simulink model "cocheaArriba"  (R2024a)
settings: Solver=VariableStepAuto  StartTime=0.0  StopTime=365*4  RelTol=1e-3
settings Model: Creator=gerar  LastModifiedBy=gerar

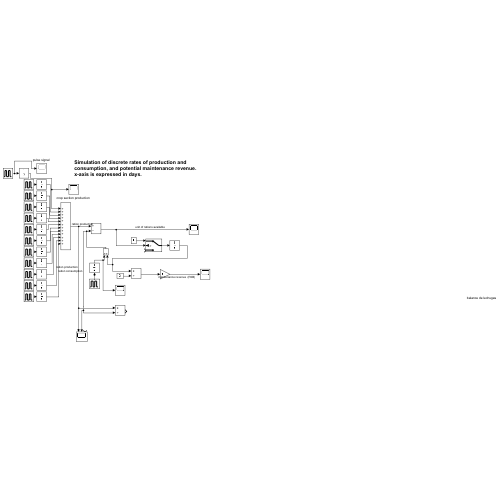
[thumbnail: Simulink's stored preview of the top-level diagram]
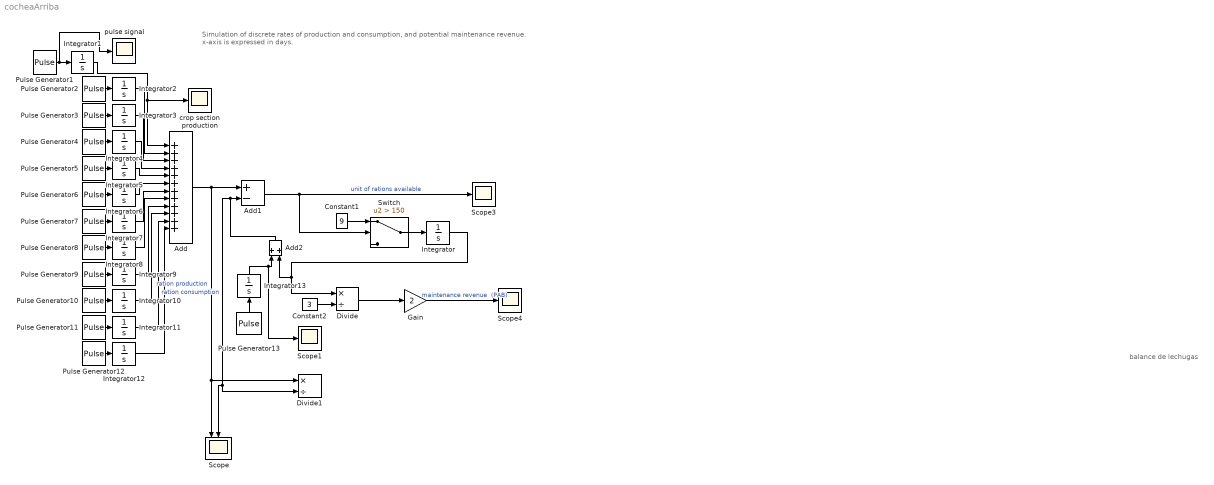
== system cocheaArriba ==
  note: Simulation of discrete rates of production and consumption, and potential maintenance revenue. x-axis is expressed in days.
  note: balance de lechugas
  Add : Sum  Inputs=++++++++++++
  Add1 : Sum  Inputs=+-
  Add2 : Sum
  Constant1 : Constant  Value=9
  Constant2 : Constant  Value=3
  Divide : Product  Inputs=*/
  Divide1 : Product  Inputs=*/
  Gain : Gain  Gain=2
  Integrator{,1..13} (14 alike) : Integrator
  Pulse Generator1 : DiscretePulseGenerator  PulseType=Time based  Amplitude=31  Period=37  PulseWidth=2.703  PhaseDelay=37
  Pulse Generator10 : DiscretePulseGenerator  PulseType=Time based  Amplitude=31  Period=37  PulseWidth=2.703  PhaseDelay=21+37
  Pulse Generator11 : DiscretePulseGenerator  PulseType=Time based  Amplitude=31  Period=37  PulseWidth=2.703  PhaseDelay=23+37
  Pulse Generator12 : DiscretePulseGenerator  PulseType=Time based  Amplitude=31  Period=37  PulseWidth=2.703  PhaseDelay=25+37
  Pulse Generator13 : DiscretePulseGenerator  PulseType=Time based  Amplitude=65  Period=7  PulseWidth=14.3  PhaseDelay=74
  Pulse Generator2 : DiscretePulseGenerator  PulseType=Time based  Amplitude=31  Period=37  PulseWidth=2.703  PhaseDelay=2+37
  Pulse Generator3 : DiscretePulseGenerator  PulseType=Time based  Amplitude=31  Period=37  PulseWidth=2.703  PhaseDelay=4+37
  Pulse Generator4 : DiscretePulseGenerator  PulseType=Time based  Amplitude=31  Period=37  PulseWidth=2.703  PhaseDelay=7+37
  Pulse Generator5 : DiscretePulseGenerator  PulseType=Time based  Amplitude=31  Period=37  PulseWidth=2.703  PhaseDelay=9+37
  Pulse Generator6 : DiscretePulseGenerator  PulseType=Time based  Amplitude=31  Period=37  PulseWidth=2.703  PhaseDelay=11+37
  Pulse Generator7 : DiscretePulseGenerator  PulseType=Time based  Amplitude=31  Period=37  PulseWidth=2.703  PhaseDelay=14+37
  Pulse Generator8 : DiscretePulseGenerator  PulseType=Time based  Amplitude=31  Period=37  PulseWidth=2.703  PhaseDelay=16+37
  Pulse Generator9 : DiscretePulseGenerator  PulseType=Time based  Amplitude=31  Period=37  PulseWidth=2.703  PhaseDelay=18+37
  Scope : Scope  NumInputPorts=3
  Scope1 : Scope
  Scope3 : Scope
  Scope4 : Scope
  Switch : Switch  Criteria=u2 > Threshold  Threshold=150  SaturateOnIntegerOverflow=off  InputSameDT=off
  "crop section production " : Scope
  "pulse signal " : Scope
  wires:
  Pulse Generator13/1 -> Integrator13/1
  Switch/1 -> Integrator/1
  Integrator/1 -> Add2/2, Divide/1
  Constant2/1 -> Divide/2
  Divide/1 -> Gain/1
  Gain/1 -> Scope4/1  "maintenance revenue  (PAB)"
  Pulse Generator1/1 -> "pulse signal "/1, Integrator1/1
  Pulse Generator2/1 -> Integrator2/1
  Pulse Generator3/1 -> Integrator3/1
  Pulse Generator4/1 -> Integrator4/1
  Pulse Generator5/1 -> Integrator5/1
  Pulse Generator6/1 -> Integrator6/1
  Pulse Generator7/1 -> Integrator7/1
  Pulse Generator8/1 -> Integrator8/1
  Pulse Generator9/1 -> Integrator9/1
  Pulse Generator10/1 -> Integrator10/1
  Pulse Generator11/1 -> Integrator11/1
  Pulse Generator12/1 -> Integrator12/1
  Integrator12/1 -> Add/12
  Integrator11/1 -> Add/11
  Integrator10/1 -> Add/10
  Integrator9/1 -> Add/9
  Integrator8/1 -> Add/8
  Integrator7/1 -> Add/7
  Integrator6/1 -> Add/6
  Integrator5/1 -> Add/5
  Integrator4/1 -> Add/4
  Integrator3/1 -> Add/3
  Integrator2/1 -> Add/2
  Integrator1/1 -> Add/1, "crop section production "/1
  Constant1/1 -> Switch/1
  Add/1 -> Add1/1, Divide1/1, Scope/1  "ration production"
  Add1/1 -> Switch/2, Scope3/1  "unit of rations available"
  Integrator13/1 -> Scope1/1, Add2/1
  Add2/1 -> Divide1/2, Scope/2, Add1/2  "ration consumption"
